simulink model "pfb_legacy"  (Simulink 6.2)
settings: Solver=ode45  StartTime=0.0  StopTime=40000  RelTol=1e-3
undefined symbols (not defined in the file): BEE2_usr
libraries: xbsIndex_r3 x189, xps_library x42, adcscope_lib x6, pfb_library x3, fft_library x3, correlator_library x3
(part 1 of 2)
settings Model: LastModifiedBy=lspitler
settings DebuggingCC: SolverPrmCheckMsg=warning

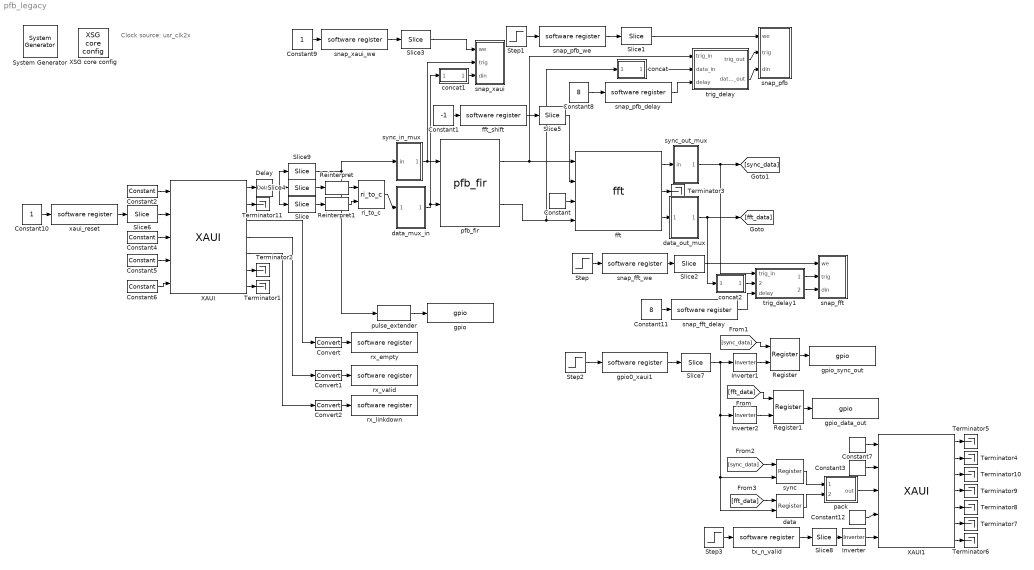
== system pfb_legacy ==
  note: Clock source: usr_clk2x
  " System Generator" : xbsIndex_r3/ System Generator  Tag=genX  xilinxfamily=Virtex2P  part=xc2vp70  speed=-7  package=ff1704  synthesis_tool=XST  directory=./pfb_legacy/sysgen  testbench=off  simulink_period=1  sysclk_period=5  incr_netlist=off  trim_vbits=Everywhere in SubSystem  dbl_ovrd=According to Block Masks  core_generation=According to Block Masks  run_coregen=off  deprecated_control=off  eval_field=0
      settings: AttributesFormatString=System\nGenerator
  Constant : xbsIndex_r3/Constant  const=0  equ=P=C  arith_type=Unsigned  n_bits=36  bin_pt=0  opselect=C  inp2=PCIN>>17  opr=+  inp1=P  carry=CIN  iostate=0  explicit_period=on  period=1  dbl_ovrd=off
  Constant1 : Constant  Value=-1
  Constant10 : Constant
  Constant11 : Constant  Value=8
  Constant12 : xbsIndex_r3/Constant  const=0  equ=P=C  arith_type=Unsigned  n_bits=4  bin_pt=0  opselect=C  inp2=PCIN>>17  opr=+  inp1=P  carry=CIN  iostate=0  explicit_period=on  period=1  dbl_ovrd=off
  Constant2 : xbsIndex_r3/Constant  const=1  equ=P=C  arith_type=Boolean  n_bits=1  bin_pt=0  opselect=C  inp2=PCIN>>17  opr=+  inp1=P  carry=CIN  iostate=0  explicit_period=on  period=1  dbl_ovrd=off
  Constant3 : xbsIndex_r3/Constant  const=0  equ=P=C  arith_type=Boolean  n_bits=36  bin_pt=0  opselect=C  inp2=PCIN>>17  opr=+  inp1=P  carry=CIN  iostate=0  explicit_period=on  period=1  dbl_ovrd=off
  Constant4 : xbsIndex_r3/Constant  const=0  equ=P=C  arith_type=Unsigned  n_bits=32  bin_pt=0  opselect=C  inp2=PCIN>>17  opr=+  inp1=P  carry=CIN  iostate=0  explicit_period=on  period=1  dbl_ovrd=off
  Constant5 : xbsIndex_r3/Constant  const=0  equ=P=C  arith_type=Unsigned  n_bits=4  bin_pt=0  opselect=C  inp2=PCIN>>17  opr=+  inp1=P  carry=CIN  iostate=0  explicit_period=on  period=1  dbl_ovrd=off
  Constant6 : xbsIndex_r3/Constant  const=0  equ=P=C  arith_type=Boolean  n_bits=1  bin_pt=0  opselect=C  inp2=PCIN>>17  opr=+  inp1=P  carry=CIN  iostate=0  explicit_period=on  period=1  dbl_ovrd=off
  Constant7 : xbsIndex_r3/Constant  const=1  equ=P=C  arith_type=Boolean  n_bits=36  bin_pt=0  opselect=C  inp2=PCIN>>17  opr=+  inp1=P  carry=CIN  iostate=0  explicit_period=on  period=1  dbl_ovrd=off
  Constant8 : Constant  Value=8
  Constant9 : Constant
  Convert : xbsIndex_r3/Convert  arith_type=Unsigned  n_bits=32  bin_pt=0  quantization=Truncate  overflow=Wrap  latency=0  explicit_period=on  period=1  dbl_ovrd=off  show_param=off  inserted_by_tool=off  pipeline=off
      settings: xl_area=[0, 0, 0, 0, 0, 0, 0]
  Convert1 : xbsIndex_r3/Convert  arith_type=Unsigned  n_bits=32  bin_pt=0  quantization=Truncate  overflow=Wrap  latency=0  explicit_period=on  period=1  dbl_ovrd=off  show_param=off  inserted_by_tool=off  pipeline=off
      settings: xl_area=[0, 0, 0, 0, 0, 0, 0]
  Convert2 : xbsIndex_r3/Convert  arith_type=Unsigned  n_bits=32  bin_pt=0  quantization=Truncate  overflow=Wrap  latency=0  explicit_period=on  period=1  dbl_ovrd=off  show_param=off  inserted_by_tool=off  pipeline=off
      settings: xl_area=[0, 0, 0, 0, 0, 0, 0]
  Delay : xbsIndex_r3/Delay  latency=1  reg_retiming=off  explicit_period=on  period=1  en=off  accept_only_valid=off  init_zero=on  dbl_ovrd=off  show_param=off
      settings: xl_area=[0, 0, 0, 0, 0, 0, 0]
  Inverter : xbsIndex_r3/Inverter  latency=0  explicit_period=off  period=1  en=off  dbl_ovrd=off  show_param=off
      settings: xl_area=[0, 0, 0, 0, 0, 0, 0]
  Inverter1 : xbsIndex_r3/Inverter  latency=0  explicit_period=off  period=1  en=off  dbl_ovrd=off  show_param=off
      settings: xl_area=[0, 0, 0, 0, 0, 0, 0]
  Inverter2 : xbsIndex_r3/Inverter  latency=0  explicit_period=off  period=1  en=off  dbl_ovrd=off  show_param=off
      settings: xl_area=[0, 0, 0, 0, 0, 0, 0]
  Register : xbsIndex_r3/Register  init=0  reg_only_valid=off  explicit_period=off  period=1  rst=off  en=on  out_en=off  dbl_ovrd=off  show_param=off
      settings: xl_area=[0, 0, 0, 0, 0, 0, 0]
  Register1 : xbsIndex_r3/Register  init=0  reg_only_valid=off  explicit_period=off  period=1  rst=off  en=on  out_en=off  dbl_ovrd=off  show_param=off
      settings: xl_area=[0, 0, 0, 0, 0, 0, 0]
  Reinterpret : xbsIndex_r3/Reinterpret  force_arith_type=on  arith_type="Signed  (2's comp)"  force_bin_pt=on  bin_pt=14  force_valid=on
  Reinterpret1 : xbsIndex_r3/Reinterpret  force_arith_type=on  arith_type="Signed  (2's comp)"  force_bin_pt=on  bin_pt=14  force_valid=on
  Slice : xbsIndex_r3/Slice  mode=Lower Bit Location + Width  nbits=15  bit1=0  base1=MSB of Input  bit0=0  base0=LSB of Input  boolean_output=off  explicit_period=on  period=1  dbl_ovrd=off
  Slice{1..3,6..8} (6 alike) : xbsIndex_r3/Slice  mode=Lower Bit Location + Width  nbits=1  bit1=0  base1=MSB of Input  bit0=0  base0=LSB of Input  boolean_output=on  explicit_period=on  period=1  dbl_ovrd=off
  Slice4 : xbsIndex_r3/Slice  mode=Lower Bit Location + Width  nbits=15  bit1=0  base1=MSB of Input  bit0=15  base0=LSB of Input  boolean_output=off  explicit_period=on  period=1  dbl_ovrd=off
  Slice5 : xbsIndex_r3/Slice  mode=Lower Bit Location + Width  nbits=12  bit1=0  base1=MSB of Input  bit0=0  base0=LSB of Input  boolean_output=off  explicit_period=off  period=1  dbl_ovrd=off
  Slice9 : xbsIndex_r3/Slice  mode=Lower Bit Location + Width  nbits=1  bit1=0  base1=MSB of Input  bit0=30  base0=LSB of Input  boolean_output=on  explicit_period=on  period=1  dbl_ovrd=off
  Step{,1..3} (4 alike) : Step  SampleTime=0
  Terminator{1..11} (11 alike) : Terminator
  XAUI : xps_library/XAUI  Tag=xps:xaui  demux=2  port=BEE2_usr:0  show_param=off  pre_emph=3  swing=800
  XAUI1 : xps_library/XAUI  Tag=xps:xaui  demux=2  port=BEE2_usr:1  show_param=off  pre_emph=3  swing=800
  XSG core config : xps_library/XSG core config  Tag=xps:xsg  hw_sys=BEE2_usr  ibob_linux=off  clk_src=usr_clk2x  gpio_clk_io_group=iBOB:sma  gpio_clk_bit_index=0  clk_rate=200  sample_period=1  synthesis_tool=XST  mpc_type=powerpc405
  concat : Subsystem
  concat1 : Subsystem
  concat2 : Subsystem
  data : xbsIndex_r3/Register  init=0  reg_only_valid=off  explicit_period=off  period=1  rst=off  en=on  out_en=off  dbl_ovrd=off  show_param=off
      settings: xl_area=[0, 0, 0, 0, 0, 0, 0]
  data_mux_in : Subsystem
  data_out_mux : Subsystem
  fft : fft_library/fft  FFTSize=12  BitWidth=18  n_inputs=0  quantization=Truncate  overflow=Wrap  add_latency=3  mult_latency=4  bram_latency=3
  fft_shift : xps_library/software register  Tag=xps:sw_reg  io_dir=From Processor  arith_type=Unsigned  bitwidth=32  bin_pt=0  sample_period=1  gw_name=pfb_legacy_fft_shift_user_data_out
  gpio : xps_library/gpio  Tag=xps:gpio  io_group=BEE2_usr:led  io_dir=out  arith_type=Boolean  bitwidth=1  bin_pt=0  bit_index=0  sample_period=1  use_single_ended=off  use_ddr=off  reg_iob=on  reg_clk_phase=0  termination=None
  gpio0_xaui1 : xps_library/software register  Tag=xps:sw_reg  io_dir=From Processor  arith_type=Unsigned  bitwidth=32  bin_pt=0  sample_period=1  gw_name=pfb_legacy_gpio0_xaui1_user_data_out
  gpio_data_out : xps_library/gpio  Tag=xps:gpio  io_group=BEE2_usr:leftlink  io_dir=out  arith_type=Unsigned  bitwidth=36  bin_pt=0  bit_index=[0:35]  sample_period=1  use_single_ended=off  use_ddr=off  reg_iob=on  reg_clk_phase=0  termination=None
  gpio_sync_out : xps_library/gpio  Tag=xps:gpio  io_group=BEE2_usr:leftlink  io_dir=out  arith_type=Boolean  bitwidth=1  bin_pt=0  bit_index=36  sample_period=1  use_single_ended=off  use_ddr=off  reg_iob=on  reg_clk_phase=0  termination=None
  pack : Subsystem
  pfb_fir : pfb_library/pfb_fir  PFBSize=12  TotalTaps=4  WindowType=hamming  n_inputs=0  MakeBiplex=off  BitWidthIn=15  BitWidthOut=18  CoeffBitWidth=8  CoeffDistMem=off  add_latency=2  mult_latency=3  bram_latency=3  quantization=Truncate  fwidth=1
      link override pol1_in1_first_tap/sync_delay/Constant: equ=P=C
      link override pol1_in1_first_tap/sync_delay/Constant1: equ=P=C
      link override pol1_in1_first_tap/sync_delay/Constant2: equ=P=C
      link override pol1_in1_first_tap/sync_delay/Constant3: equ=P=C
      link override pol1_in1_last_tap/pfb_add_tree/convert1: arith_type="Signed  (2's comp)"  n_bits=BitWidthOut  bin_pt=BitWidthOut-1  quantization=Truncate  overflow=Saturate  latency=add_latency  pipeline=on
      link override pol1_in1_last_tap/pfb_add_tree/convert2: arith_type="Signed  (2's comp)"  n_bits=BitWidthOut  bin_pt=BitWidthOut-1  quantization="Round  (unbiased: +/- Inf)"  overflow=Saturate  latency=add_latency  pipeline=on
      link override pol1_in1_tap2/sync_delay/Constant: equ=P=C
      link override pol1_in1_tap2/sync_delay/Constant1: equ=P=C
      link override pol1_in1_tap2/sync_delay/Constant2: equ=P=C
      link override pol1_in1_tap2/sync_delay/Constant3: equ=P=C
      link override pol1_in1_tap3/sync_delay/Constant: equ=P=C
      link override pol1_in1_tap3/sync_delay/Constant1: equ=P=C
      link override pol1_in1_tap3/sync_delay/Constant2: equ=P=C
      link override pol1_in1_tap3/sync_delay/Constant3: equ=P=C
      link override pol1_in2_first_tap/sync_delay/Constant: equ=P=C
      link override pol1_in2_first_tap/sync_delay/Constant1: equ=P=C
      link override pol1_in2_first_tap/sync_delay/Constant2: equ=P=C
      link override pol1_in2_first_tap/sync_delay/Constant3: equ=P=C
  pulse_extender : adcscope_lib/pulse_extender  pulse_len=2^12-1
  ri_to_c : fft_library/ri_to_c  likes_cookies=off
  rx_empty : xps_library/software register  Tag=xps:sw_reg  io_dir=To Processor  arith_type=Unsigned  bitwidth=32  bin_pt=0  sample_period=1  gw_name=pfb_legacy_rx_empty_user_data_in
  rx_linkdown : xps_library/software register  Tag=xps:sw_reg  io_dir=To Processor  arith_type=Unsigned  bitwidth=32  bin_pt=0  sample_period=1  gw_name=pfb_legacy_rx_linkdown_user_data_in
  rx_valid : xps_library/software register  Tag=xps:sw_reg  io_dir=To Processor  arith_type=Unsigned  bitwidth=32  bin_pt=0  sample_period=1  gw_name=pfb_legacy_rx_valid_user_data_in
  snap_fft : Subsystem  mask{nsamples=12}
      mask prompts: nsamples "number of samples (2^?)"
  snap_fft_delay : xps_library/software register  Tag=xps:sw_reg  io_dir=From Processor  arith_type=Unsigned  bitwidth=32  bin_pt=0  sample_period=1  gw_name=pfb_legacy_snap_fft_delay_user_data_out
  snap_fft_we : xps_library/software register  Tag=xps:sw_reg  io_dir=From Processor  arith_type=Unsigned  bitwidth=32  bin_pt=0  sample_period=1  gw_name=pfb_legacy_snap_fft_we_user_data_out
  snap_pfb : Subsystem  mask{nsamples=12}
      mask prompts: nsamples "number of samples (2^?)"
  snap_pfb_delay : xps_library/software register  Tag=xps:sw_reg  io_dir=From Processor  arith_type=Unsigned  bitwidth=32  bin_pt=0  sample_period=1  gw_name=pfb_legacy_snap_pfb_delay_user_data_out
  snap_pfb_we : xps_library/software register  Tag=xps:sw_reg  io_dir=From Processor  arith_type=Unsigned  bitwidth=32  bin_pt=0  sample_period=1  gw_name=pfb_legacy_snap_pfb_we_user_data_out
  snap_xaui : Subsystem  mask{nsamples=12}
      mask prompts: nsamples "number of samples (2^?)"
  snap_xaui_we : xps_library/software register  Tag=xps:sw_reg  io_dir=From Processor  arith_type=Unsigned  bitwidth=32  bin_pt=0  sample_period=1  gw_name=pfb_legacy_snap_xaui_we_user_data_out
  sync : xbsIndex_r3/Register  init=0  reg_only_valid=off  explicit_period=off  period=1  rst=off  en=on  out_en=off  dbl_ovrd=off  show_param=off
      settings: xl_area=[0, 0, 0, 0, 0, 0, 0]
  sync_in_mux : Subsystem
  sync_out_mux : Subsystem
  trig_delay : Subsystem
  trig_delay1 : Subsystem
  tx_n_valid : xps_library/software register  Tag=xps:sw_reg  io_dir=From Processor  arith_type=Unsigned  bitwidth=32  bin_pt=0  sample_period=1  gw_name=pfb_legacy_tx_n_valid_user_data_out
  xaui_reset : xps_library/software register  Tag=xps:sw_reg  io_dir=From Processor  arith_type=Unsigned  bitwidth=32  bin_pt=0  sample_period=1  gw_name=pfb_legacy_xaui_reset_user_data_out
  wires:
  XAUI/1 -> Delay/1
  XAUI/4 -> Convert1/1
  pfb_fir/1 -> trig_delay/1(trig_in), fft/1
  Constant2/1 -> XAUI/1
  Constant4/1 -> XAUI/3
  Constant5/1 -> XAUI/4
  Constant6/1 -> XAUI/5
  XAUI/7 -> Terminator1/1
  XAUI/6 -> Terminator2/1
  Convert/1 -> rx_empty/1
  Convert1/1 -> rx_valid/1
  Convert2/1 -> rx_linkdown/1
  XAUI/3 -> Convert/1
  XAUI/5 -> Convert2/1
  Constant/1 -> fft/3
  data_mux_in/1(Out2) -> pfb_fir/2, concat1/1(In1)
  pfb_fir/2 -> fft/4, concat/1(In1)
  fft/2 -> Terminator3/1
  fft/3 -> data_out_mux/1(In1)
  fft/1 -> sync_out_mux/1(in)
  sync_out_mux/1(out) -> trig_delay1/1(trig_in), [sync_data]
  data_out_mux/1(Out2) -> concat2/1(In1), [fft_data]
  snap_fft_we/1 -> Slice2/1
  Step/1 -> snap_fft_we/1
  snap_xaui_we/1 -> Slice3/1
  Slice3/1 -> snap_xaui/1(we)
  Constant9/1 -> snap_xaui_we/1
  Slice2/1 -> snap_fft/1(we)
  fft_shift/1 -> Slice5/1
  Constant1/1 -> fft_shift/1
  sync_in_mux/1(out) -> pfb_fir/1, snap_xaui/2(trig)
  Slice5/1 -> fft/2
  xaui_reset/1 -> Slice6/1
  Constant10/1 -> xaui_reset/1
  Slice6/1 -> XAUI/2
  concat1/1(Out1) -> snap_xaui/3(din)
  snap_pfb_we/1 -> Slice1/1
  Step1/1 -> snap_pfb_we/1
  Slice1/1 -> snap_pfb/1(we)
  pulse_extender/1 -> gpio/1
  Constant3/1 -> XAUI1/2
  Constant7/1 -> XAUI1/1
  tx_n_valid/1 -> Slice8/1
  Step3/1 -> tx_n_valid/1
  Slice8/1 -> Inverter/1
  Inverter/1 -> XAUI1/5
  XAUI1/1 -> Terminator5/1
  XAUI1/2 -> Terminator4/1
  XAUI1/6 -> Terminator7/1
  XAUI1/7 -> Terminator6/1
  XAUI1/3 -> Terminator10/1
  XAUI1/4 -> Terminator9/1
  XAUI1/5 -> Terminator8/1
  Constant8/1 -> snap_pfb_delay/1
  snap_pfb_delay/1 -> trig_delay/3(delay)
  concat/1(Out1) -> trig_delay/2(data_in)
  trig_delay/1(trig_out) -> snap_pfb/2(trig)
  trig_delay/2(data_out) -> snap_pfb/3(din)
  snap_fft_delay/1 -> trig_delay1/3(delay)
  concat2/1(Out1) -> trig_delay1/2(data_in)
  trig_delay1/1(trig_out) -> snap_fft/2(trig)
  trig_delay1/2(data_out) -> snap_fft/3(din)
  Constant11/1 -> snap_fft_delay/1
  Delay/1 -> Slice9/1, Slice4/1, Slice/1
  XAUI/2 -> Terminator11/1
  Slice9/1 -> sync_in_mux/1(in), pulse_extender/1
  Slice4/1 -> Reinterpret/1
  Slice/1 -> Reinterpret1/1
  Reinterpret/1 -> ri_to_c/1
  Reinterpret1/1 -> ri_to_c/2
  ri_to_c/1 -> data_mux_in/1(In1)
  Register/1 -> gpio_sync_out/1
  gpio0_xaui1/1 -> Slice7/1
  Slice7/1 -> Inverter1/1, Inverter2/1, sync/2, data/2
  Register1/1 -> gpio_data_out/1
  Inverter1/1 -> Register/2
  Step2/1 -> gpio0_xaui1/1
  Inverter2/1 -> Register1/2
  [fft_data] -> Register1/1
  [sync_data] -> Register/1
  pack/1(out) -> XAUI1/3
  sync/1 -> pack/1(sync)
  data/1 -> pack/2(data)
  [sync_data] -> sync/1
  [fft_data] -> data/1
  Constant12/1 -> XAUI1/4

== system pfb_legacy/concat ==
  In1 : Inport  Orientation=down  Port=1  LatchInput=off
  Concat : xbsIndex_r3/Concat  num_inputs=4  explicit_period=on  period=1  dbl_ovrd=off
  Constant7 : xbsIndex_r3/Constant  const=0  equ=P=C  arith_type=Unsigned  n_bits=14  bin_pt=0  opselect=C  inp2=PCIN>>17  opr=+  inp1=P  carry=CIN  iostate=0  explicit_period=on  period=1  dbl_ovrd=off
  Constant8 : xbsIndex_r3/Constant  const=0  equ=P=C  arith_type=Unsigned  n_bits=14  bin_pt=0  opselect=C  inp2=PCIN>>17  opr=+  inp1=P  carry=CIN  iostate=0  explicit_period=on  period=1  dbl_ovrd=off
  Slice : xbsIndex_r3/Slice  mode=Upper Bit Location + Width  nbits=18  bit1=0  base1=MSB of Input  bit0=0  base0=LSB of Input  boolean_output=off  explicit_period=on  period=1  dbl_ovrd=off
  Slice1 : xbsIndex_r3/Slice  mode=Lower Bit Location + Width  nbits=18  bit1=0  base1=MSB of Input  bit0=0  base0=LSB of Input  boolean_output=off  explicit_period=on  period=1  dbl_ovrd=off
  Out1 : Outport
  wires:
  Slice/1 -> Concat/2
  Slice1/1 -> Concat/4
  Constant7/1 -> Concat/1
  Constant8/1 -> Concat/3
  In1/1 -> Slice/1, Slice1/1
  Concat/1 -> Out1/1

== system pfb_legacy/concat1 ==
  In1 : Inport  Port=1  LatchInput=off
  Concat1 : xbsIndex_r3/Concat  num_inputs=4  explicit_period=on  period=1  dbl_ovrd=off
  Constant11 : xbsIndex_r3/Constant  const=0  equ=P=C  arith_type=Unsigned  n_bits=16  bin_pt=0  opselect=C  inp2=PCIN>>17  opr=+  inp1=P  carry=CIN  iostate=0  explicit_period=on  period=1  dbl_ovrd=off
  Constant3 : xbsIndex_r3/Constant  const=0  equ=P=C  arith_type=Unsigned  n_bits=16  bin_pt=0  opselect=C  inp2=PCIN>>17  opr=+  inp1=P  carry=CIN  iostate=0  explicit_period=on  period=1  dbl_ovrd=off
  Slice7 : xbsIndex_r3/Slice  mode=Upper Bit Location + Width  nbits=16  bit1=0  base1=MSB of Input  bit0=0  base0=LSB of Input  boolean_output=off  explicit_period=on  period=1  dbl_ovrd=off
  Slice8 : xbsIndex_r3/Slice  mode=Lower Bit Location + Width  nbits=16  bit1=0  base1=MSB of Input  bit0=0  base0=LSB of Input  boolean_output=off  explicit_period=on  period=1  dbl_ovrd=off
  Out1 : Outport
  wires:
  Slice7/1 -> Concat1/2
  Slice8/1 -> Concat1/4
  Constant3/1 -> Concat1/1
  Constant11/1 -> Concat1/3
  In1/1 -> Slice7/1, Slice8/1
  Concat1/1 -> Out1/1

== system pfb_legacy/concat2 ==
  In1 : Inport  Orientation=down  Port=1  LatchInput=off
  Concat : xbsIndex_r3/Concat  num_inputs=4  explicit_period=on  period=1  dbl_ovrd=off
  Constant7 : xbsIndex_r3/Constant  const=0  equ=P=C  arith_type=Unsigned  n_bits=14  bin_pt=0  opselect=C  inp2=PCIN>>17  opr=+  inp1=P  carry=CIN  iostate=0  explicit_period=on  period=1  dbl_ovrd=off
  Constant8 : xbsIndex_r3/Constant  const=0  equ=P=C  arith_type=Unsigned  n_bits=14  bin_pt=0  opselect=C  inp2=PCIN>>17  opr=+  inp1=P  carry=CIN  iostate=0  explicit_period=on  period=1  dbl_ovrd=off
  Slice : xbsIndex_r3/Slice  mode=Upper Bit Location + Width  nbits=18  bit1=0  base1=MSB of Input  bit0=0  base0=LSB of Input  boolean_output=off  explicit_period=on  period=1  dbl_ovrd=off
  Slice1 : xbsIndex_r3/Slice  mode=Lower Bit Location + Width  nbits=18  bit1=0  base1=MSB of Input  bit0=0  base0=LSB of Input  boolean_output=off  explicit_period=on  period=1  dbl_ovrd=off
  Out1 : Outport
  wires:
  Slice/1 -> Concat/2
  Slice1/1 -> Concat/4
  Constant7/1 -> Concat/1
  Constant8/1 -> Concat/3
  In1/1 -> Slice/1, Slice1/1
  Concat/1 -> Out1/1

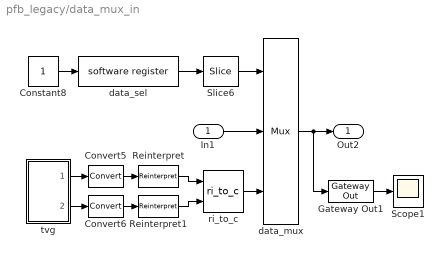
== system pfb_legacy/data_mux_in ==
  In1 : Inport  Port=1  LatchInput=off
  Constant8 : Constant
  Convert5 : xbsIndex_r3/Convert  arith_type="Signed  (2's comp)"  n_bits=15  bin_pt=0  quantization=Truncate  overflow=Wrap  latency=0  explicit_period=on  period=1  dbl_ovrd=off  show_param=off  inserted_by_tool=off  pipeline=off
      settings: xl_area=[0, 0, 0, 0, 0, 0, 0]
  Convert6 : xbsIndex_r3/Convert  arith_type="Signed  (2's comp)"  n_bits=15  bin_pt=0  quantization=Truncate  overflow=Wrap  latency=0  explicit_period=on  period=1  dbl_ovrd=off  show_param=off  inserted_by_tool=off  pipeline=off
      settings: xl_area=[0, 0, 0, 0, 0, 0, 0]
  Gateway Out1 : xbsIndex_r3/Gateway Out  output_type=Double  nbits=8  bin_pt=6  arith_type=Boolean  quantization=Truncate  overflow=Wrap  hdl_port=on  timing_constraint=None  locs_specified=off  LOCs={}  needs_fixed_name=off  show_param=off
      settings: xl_area=[0, 0, 0, 0, 0, 0, 0]
  Reinterpret : xbsIndex_r3/Reinterpret  force_arith_type=off  arith_type=Unsigned  force_bin_pt=on  bin_pt=14  force_valid=on
  Reinterpret1 : xbsIndex_r3/Reinterpret  force_arith_type=off  arith_type=Unsigned  force_bin_pt=on  bin_pt=14  force_valid=on
  Scope1 : Scope
      settings: SaveName=ScopeData5
  Slice6 : xbsIndex_r3/Slice  mode=Lower Bit Location + Width  nbits=1  bit1=0  base1=MSB of Input  bit0=0  base0=LSB of Input  boolean_output=off  explicit_period=off  period=1  dbl_ovrd=off
  data_mux : xbsIndex_r3/Mux  inputs=2  precision=Full  arith_type="Signed  (2's comp)"  n_bits=8  bin_pt=2  quantization=Truncate  overflow=Wrap  latency=0  explicit_period=on  period=1  en=off  dbl_ovrd=off  show_param=off  mux_type=off  use_rpm=off  gen_core=off
      settings: xl_area=[0, 0, 0, 0, 0, 0, 0]
  data_sel : xps_library/software register  Tag=xps:sw_reg  io_dir=From Processor  arith_type=Unsigned  bitwidth=32  bin_pt=0  sample_period=1  gw_name=pfb_legacy_data_mux_in_data_sel_user_data_out
  ri_to_c : pfb_library/tap/ri_to_c
  tvg : Subsystem
  Out2 : Outport
  wires:
  data_sel/1 -> Slice6/1
  Constant8/1 -> data_sel/1
  Slice6/1 -> data_mux/1
  In1/1 -> data_mux/2
  data_mux/1 -> Gateway Out1/1, Out2/1
  Gateway Out1/1 -> Scope1/1
  tvg/1(re_out) -> Convert5/1
  tvg/2(im_out) -> Convert6/1
  Convert5/1 -> Reinterpret/1
  Convert6/1 -> Reinterpret1/1
  ri_to_c/1 -> data_mux/3
  Reinterpret/1 -> ri_to_c/1
  Reinterpret1/1 -> ri_to_c/2

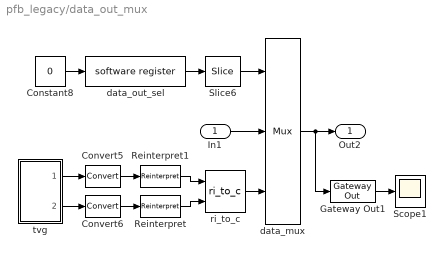
== system pfb_legacy/data_out_mux ==
  In1 : Inport  Port=1  LatchInput=off
  Constant8 : Constant  Value=0
  Convert5 : xbsIndex_r3/Convert  arith_type="Signed  (2's comp)"  n_bits=18  bin_pt=0  quantization=Truncate  overflow=Wrap  latency=0  explicit_period=on  period=1  dbl_ovrd=off  show_param=off  inserted_by_tool=off  pipeline=off
      settings: xl_area=[0, 0, 0, 0, 0, 0, 0]
  Convert6 : xbsIndex_r3/Convert  arith_type="Signed  (2's comp)"  n_bits=18  bin_pt=0  quantization=Truncate  overflow=Wrap  latency=0  explicit_period=on  period=1  dbl_ovrd=off  show_param=off  inserted_by_tool=off  pipeline=off
      settings: xl_area=[0, 0, 0, 0, 0, 0, 0]
  Gateway Out1 : xbsIndex_r3/Gateway Out  output_type=Double  nbits=8  bin_pt=6  arith_type=Boolean  quantization=Truncate  overflow=Wrap  hdl_port=on  timing_constraint=None  locs_specified=off  LOCs={}  needs_fixed_name=off  show_param=off
      settings: xl_area=[0, 0, 0, 0, 0, 0, 0]
  Reinterpret : xbsIndex_r3/Reinterpret  force_arith_type=off  arith_type=Unsigned  force_bin_pt=on  bin_pt=17  force_valid=on
  Reinterpret1 : xbsIndex_r3/Reinterpret  force_arith_type=off  arith_type=Unsigned  force_bin_pt=on  bin_pt=17  force_valid=on
  Scope1 : Scope
      settings: SaveName=ScopeData5
  Slice6 : xbsIndex_r3/Slice  mode=Lower Bit Location + Width  nbits=1  bit1=0  base1=MSB of Input  bit0=0  base0=LSB of Input  boolean_output=off  explicit_period=off  period=1  dbl_ovrd=off
  data_mux : xbsIndex_r3/Mux  inputs=2  precision=Full  arith_type="Signed  (2's comp)"  n_bits=8  bin_pt=2  quantization=Truncate  overflow=Wrap  latency=0  explicit_period=on  period=1  en=off  dbl_ovrd=off  show_param=off  mux_type=off  use_rpm=off  gen_core=off
      settings: xl_area=[0, 0, 0, 0, 0, 0, 0]
  data_out_sel : xps_library/software register  Tag=xps:sw_reg  io_dir=From Processor  arith_type=Unsigned  bitwidth=32  bin_pt=0  sample_period=1  gw_name=pfb_legacy_data_out_mux_data_out_sel_user_data_out
  ri_to_c : pfb_library/tap/ri_to_c
  tvg : Subsystem
  Out2 : Outport
  wires:
  ri_to_c/1 -> data_mux/3
  Convert6/1 -> Reinterpret/1
  tvg/2(im_out) -> Convert6/1
  tvg/1(re_out) -> Convert5/1
  Gateway Out1/1 -> Scope1/1
  data_mux/1 -> Out2/1, Gateway Out1/1
  In1/1 -> data_mux/2
  Slice6/1 -> data_mux/1
  Constant8/1 -> data_out_sel/1
  data_out_sel/1 -> Slice6/1
  Reinterpret/1 -> ri_to_c/2
  Convert5/1 -> Reinterpret1/1
  Reinterpret1/1 -> ri_to_c/1

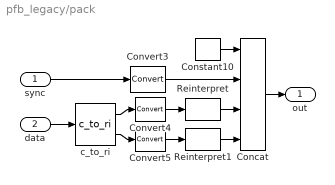
== system pfb_legacy/pack ==
  sync : Inport  Port=1  LatchInput=off
  data : Inport  Port=2  LatchInput=off
  Concat : xbsIndex_r3/Concat  num_inputs=4  explicit_period=on  period=1  dbl_ovrd=off
  Constant10 : xbsIndex_r3/Constant  const=0  equ=P=C  arith_type=Unsigned  n_bits=1  bin_pt=0  opselect=C  inp2=PCIN>>17  opr=+  inp1=P  carry=CIN  iostate=0  explicit_period=on  period=1  dbl_ovrd=off
  Convert3 : xbsIndex_r3/Convert  arith_type=Unsigned  n_bits=1  bin_pt=0  quantization=Truncate  overflow=Wrap  latency=1  explicit_period=on  period=1  dbl_ovrd=off  show_param=off  inserted_by_tool=off  pipeline=off
      settings: xl_area=[0, 0, 0, 0, 0, 0, 0]
  Convert4 : xbsIndex_r3/Convert  arith_type="Signed  (2's comp)"  n_bits=15  bin_pt=14  quantization=Truncate  overflow=Wrap  latency=1  explicit_period=on  period=1  dbl_ovrd=off  show_param=off  inserted_by_tool=off  pipeline=off
      settings: xl_area=[0, 0, 0, 0, 0, 0, 0]
  Convert5 : xbsIndex_r3/Convert  arith_type="Signed  (2's comp)"  n_bits=15  bin_pt=14  quantization=Truncate  overflow=Wrap  latency=1  explicit_period=on  period=1  dbl_ovrd=off  show_param=off  inserted_by_tool=off  pipeline=off
      settings: xl_area=[0, 0, 0, 0, 0, 0, 0]
  Reinterpret : xbsIndex_r3/Reinterpret  force_arith_type=on  arith_type=Unsigned  force_bin_pt=on  bin_pt=0  force_valid=on
  Reinterpret1 : xbsIndex_r3/Reinterpret  force_arith_type=on  arith_type=Unsigned  force_bin_pt=on  bin_pt=0  force_valid=on
  c_to_ri : fft_library/c_to_ri  BitWidth=18
  out : Outport
  wires:
  Reinterpret1/1 -> Concat/4
  Convert5/1 -> Reinterpret1/1
  data/1 -> c_to_ri/1
  Concat/1 -> out/1
  sync/1 -> Convert3/1
  Reinterpret/1 -> Concat/3
  Convert4/1 -> Reinterpret/1
  Convert3/1 -> Concat/2
  c_to_ri/2 -> Convert5/1
  c_to_ri/1 -> Convert4/1
  Constant10/1 -> Concat/1

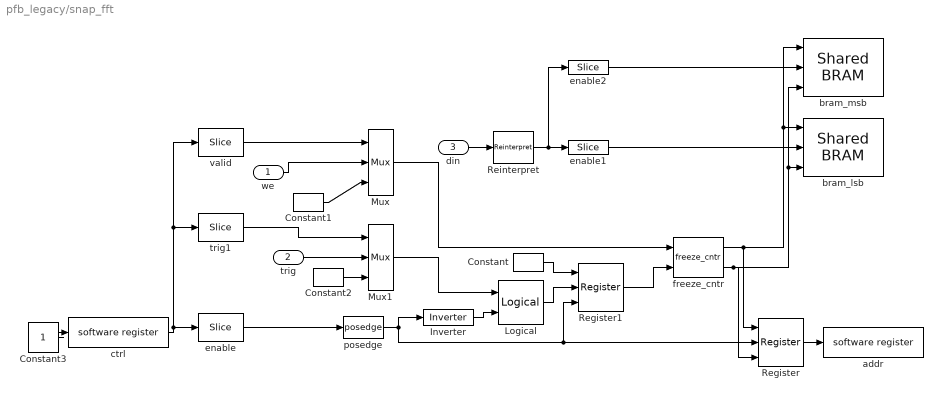
== system pfb_legacy/snap_fft ==
  we : Inport  Port=1  LatchInput=off
  trig : Inport  Port=2  LatchInput=off
  din : Inport  Port=3  LatchInput=off
  Constant : xbsIndex_r3/Constant  const=1  equ=P=C  arith_type=Boolean  n_bits=1  bin_pt=0  opselect=C  inp2=PCIN>>17  opr=+  inp1=P  carry=CIN  iostate=0  explicit_period=on  period=1  dbl_ovrd=off
  Constant1 : xbsIndex_r3/Constant  const=1  equ=P=C  arith_type=Boolean  n_bits=1  bin_pt=0  opselect=C  inp2=PCIN>>17  opr=+  inp1=P  carry=CIN  iostate=0  explicit_period=on  period=1  dbl_ovrd=off
  Constant2 : xbsIndex_r3/Constant  const=1  equ=P=C  arith_type=Boolean  n_bits=1  bin_pt=0  opselect=C  inp2=PCIN>>17  opr=+  inp1=P  carry=CIN  iostate=0  explicit_period=on  period=1  dbl_ovrd=off
  Constant3 : Constant
  Inverter : xbsIndex_r3/Inverter  latency=0  explicit_period=on  period=1  en=off  dbl_ovrd=off  show_param=off
      settings: xl_area=[0, 0, 0, 0, 0, 0, 0]
  Logical : xbsIndex_r3/Logical  logical_function=AND  inputs=2  precision=Full  arith_type=Unsigned  n_bits=8  bin_pt=2  align_bp=on  latency=0  explicit_period=off  period=1  en=off  dbl_ovrd=off  show_param=off
      settings: xl_area=[0, 0, 0, 0, 0, 0, 0]
  Mux : xbsIndex_r3/Mux  inputs=2  precision=Full  arith_type="Signed  (2's comp)"  n_bits=8  bin_pt=2  quantization=Truncate  overflow=Wrap  latency=0  explicit_period=on  period=1  en=off  dbl_ovrd=off  show_param=off  mux_type=off  use_rpm=off  gen_core=off
      settings: xl_area=[0, 0, 0, 0, 0, 0, 0]
  Mux1 : xbsIndex_r3/Mux  inputs=2  precision=Full  arith_type="Signed  (2's comp)"  n_bits=8  bin_pt=2  quantization=Truncate  overflow=Wrap  latency=0  explicit_period=on  period=1  en=off  dbl_ovrd=off  show_param=off  mux_type=off  use_rpm=off  gen_core=off
      settings: xl_area=[0, 0, 0, 0, 0, 0, 0]
  Register : xbsIndex_r3/Register  init=0  reg_only_valid=off  explicit_period=on  period=1  rst=on  en=on  out_en=off  dbl_ovrd=off  show_param=off
      settings: xl_area=[0, 0, 0, 0, 0, 0, 0]
  Register1 : xbsIndex_r3/Register  init=0  reg_only_valid=off  explicit_period=on  period=1  rst=on  en=on  out_en=off  dbl_ovrd=off  show_param=off
      settings: xl_area=[0, 0, 0, 0, 0, 0, 0]
  Reinterpret : xbsIndex_r3/Reinterpret  force_arith_type=on  arith_type=Unsigned  force_bin_pt=on  bin_pt=0  force_valid=on
  addr : xps_library/software register  Tag=xps:sw_reg  io_dir=To Processor  arith_type=Unsigned  bitwidth=32  bin_pt=0  sample_period=1  gw_name=pfb_legacy_snap_fft_addr_user_data_in
  bram_lsb : xps_library/Shared BRAM  Tag=xps:bram  arith_type=Unsigned  addr_width=nsamples  data_width=32  data_bin_pt=0  init_vals=0  sample_rate=1
  bram_msb : xps_library/Shared BRAM  Tag=xps:bram  arith_type=Unsigned  addr_width=nsamples  data_width=32  data_bin_pt=0  init_vals=0  sample_rate=1
  ctrl : xps_library/software register  Tag=xps:sw_reg  io_dir=From Processor  arith_type=Unsigned  bitwidth=32  bin_pt=0  sample_period=1  gw_name=pfb_legacy_snap_fft_ctrl_user_data_out
  enable : xbsIndex_r3/Slice  mode=Lower Bit Location + Width  nbits=1  bit1=0  base1=MSB of Input  bit0=0  base0=LSB of Input  boolean_output=on  explicit_period=on  period=1  dbl_ovrd=off
  enable1 : xbsIndex_r3/Slice  mode=Lower Bit Location + Width  nbits=32  bit1=0  base1=MSB of Input  bit0=0  base0=LSB of Input  boolean_output=off  explicit_period=on  period=1  dbl_ovrd=off
  enable2 : xbsIndex_r3/Slice  mode=Lower Bit Location + Width  nbits=32  bit1=0  base1=MSB of Input  bit0=32  base0=LSB of Input  boolean_output=off  explicit_period=on  period=1  dbl_ovrd=off
  freeze_cntr : correlator_library/freeze_cntr  CounterBits=nsamples
  posedge : adcscope_lib/posedge  Tag=Rising Edge Detector  yummy=on
  trig1 : xbsIndex_r3/Slice  mode=Lower Bit Location + Width  nbits=1  bit1=1  base1=MSB of Input  bit0=1  base0=LSB of Input  boolean_output=on  explicit_period=on  period=1  dbl_ovrd=off
  valid : xbsIndex_r3/Slice  mode=Lower Bit Location + Width  nbits=1  bit1=0  base1=MSB of Input  bit0=2  base0=LSB of Input  boolean_output=on  explicit_period=on  period=1  dbl_ovrd=off
  wires:
  Constant3/1 -> ctrl/1
  ctrl/1 -> valid/1, trig1/1, enable/1
  valid/1 -> Mux/1
  trig1/1 -> Mux1/1
  freeze_cntr/2 -> bram_msb/3, bram_lsb/3, Register/3
  freeze_cntr/1 -> Register/1, bram_msb/1, bram_lsb/1
  Mux/1 -> freeze_cntr/1
  Mux1/1 -> Logical/1
  Constant/1 -> Register1/1
  Logical/1 -> Register1/2
  Register1/1 -> freeze_cntr/2
  Inverter/1 -> Logical/2
  din/1 -> Reinterpret/1
  Constant2/1 -> Mux1/3
  Constant1/1 -> Mux/3
  trig/1 -> Mux1/2
  we/1 -> Mux/2
  Reinterpret/1 -> enable2/1, enable1/1
  enable1/1 -> bram_lsb/2
  enable2/1 -> bram_msb/2
  Register/1 -> addr/1
  posedge/1 -> Register1/3, Register/2, Inverter/1
  enable/1 -> posedge/1

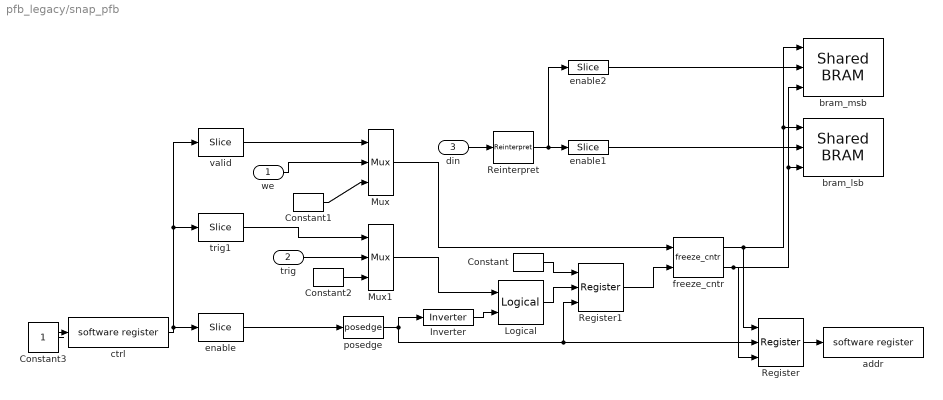
== system pfb_legacy/snap_pfb ==
  we : Inport  Port=1  LatchInput=off
  trig : Inport  Port=2  LatchInput=off
  din : Inport  Port=3  LatchInput=off
  Constant : xbsIndex_r3/Constant  const=1  equ=P=C  arith_type=Boolean  n_bits=1  bin_pt=0  opselect=C  inp2=PCIN>>17  opr=+  inp1=P  carry=CIN  iostate=0  explicit_period=on  period=1  dbl_ovrd=off
  Constant1 : xbsIndex_r3/Constant  const=1  equ=P=C  arith_type=Boolean  n_bits=1  bin_pt=0  opselect=C  inp2=PCIN>>17  opr=+  inp1=P  carry=CIN  iostate=0  explicit_period=on  period=1  dbl_ovrd=off
  Constant2 : xbsIndex_r3/Constant  const=1  equ=P=C  arith_type=Boolean  n_bits=1  bin_pt=0  opselect=C  inp2=PCIN>>17  opr=+  inp1=P  carry=CIN  iostate=0  explicit_period=on  period=1  dbl_ovrd=off
  Constant3 : Constant
  Inverter : xbsIndex_r3/Inverter  latency=0  explicit_period=on  period=1  en=off  dbl_ovrd=off  show_param=off
      settings: xl_area=[0, 0, 0, 0, 0, 0, 0]
  Logical : xbsIndex_r3/Logical  logical_function=AND  inputs=2  precision=Full  arith_type=Unsigned  n_bits=8  bin_pt=2  align_bp=on  latency=0  explicit_period=off  period=1  en=off  dbl_ovrd=off  show_param=off
      settings: xl_area=[0, 0, 0, 0, 0, 0, 0]
  Mux : xbsIndex_r3/Mux  inputs=2  precision=Full  arith_type="Signed  (2's comp)"  n_bits=8  bin_pt=2  quantization=Truncate  overflow=Wrap  latency=0  explicit_period=on  period=1  en=off  dbl_ovrd=off  show_param=off  mux_type=off  use_rpm=off  gen_core=off
      settings: xl_area=[0, 0, 0, 0, 0, 0, 0]
  Mux1 : xbsIndex_r3/Mux  inputs=2  precision=Full  arith_type="Signed  (2's comp)"  n_bits=8  bin_pt=2  quantization=Truncate  overflow=Wrap  latency=0  explicit_period=on  period=1  en=off  dbl_ovrd=off  show_param=off  mux_type=off  use_rpm=off  gen_core=off
      settings: xl_area=[0, 0, 0, 0, 0, 0, 0]
  Register : xbsIndex_r3/Register  init=0  reg_only_valid=off  explicit_period=on  period=1  rst=on  en=on  out_en=off  dbl_ovrd=off  show_param=off
      settings: xl_area=[0, 0, 0, 0, 0, 0, 0]
  Register1 : xbsIndex_r3/Register  init=0  reg_only_valid=off  explicit_period=on  period=1  rst=on  en=on  out_en=off  dbl_ovrd=off  show_param=off
      settings: xl_area=[0, 0, 0, 0, 0, 0, 0]
  Reinterpret : xbsIndex_r3/Reinterpret  force_arith_type=on  arith_type=Unsigned  force_bin_pt=on  bin_pt=0  force_valid=on
  addr : xps_library/software register  Tag=xps:sw_reg  io_dir=To Processor  arith_type=Unsigned  bitwidth=32  bin_pt=0  sample_period=1  gw_name=pfb_legacy_snap_pfb_addr_user_data_in
  bram_lsb : xps_library/Shared BRAM  Tag=xps:bram  arith_type=Unsigned  addr_width=nsamples  data_width=32  data_bin_pt=0  init_vals=0  sample_rate=1
  bram_msb : xps_library/Shared BRAM  Tag=xps:bram  arith_type=Unsigned  addr_width=nsamples  data_width=32  data_bin_pt=0  init_vals=0  sample_rate=1
  ctrl : xps_library/software register  Tag=xps:sw_reg  io_dir=From Processor  arith_type=Unsigned  bitwidth=32  bin_pt=0  sample_period=1  gw_name=pfb_legacy_snap_pfb_ctrl_user_data_out
  enable : xbsIndex_r3/Slice  mode=Lower Bit Location + Width  nbits=1  bit1=0  base1=MSB of Input  bit0=0  base0=LSB of Input  boolean_output=on  explicit_period=on  period=1  dbl_ovrd=off
  enable1 : xbsIndex_r3/Slice  mode=Lower Bit Location + Width  nbits=32  bit1=0  base1=MSB of Input  bit0=0  base0=LSB of Input  boolean_output=off  explicit_period=on  period=1  dbl_ovrd=off
  enable2 : xbsIndex_r3/Slice  mode=Lower Bit Location + Width  nbits=32  bit1=0  base1=MSB of Input  bit0=32  base0=LSB of Input  boolean_output=off  explicit_period=on  period=1  dbl_ovrd=off
  freeze_cntr : correlator_library/freeze_cntr  CounterBits=nsamples
  posedge : adcscope_lib/posedge  Tag=Rising Edge Detector  yummy=on
  trig1 : xbsIndex_r3/Slice  mode=Lower Bit Location + Width  nbits=1  bit1=1  base1=MSB of Input  bit0=1  base0=LSB of Input  boolean_output=on  explicit_period=on  period=1  dbl_ovrd=off
  valid : xbsIndex_r3/Slice  mode=Lower Bit Location + Width  nbits=1  bit1=0  base1=MSB of Input  bit0=2  base0=LSB of Input  boolean_output=on  explicit_period=on  period=1  dbl_ovrd=off
  wires:
  Constant3/1 -> ctrl/1
  ctrl/1 -> valid/1, trig1/1, enable/1
  valid/1 -> Mux/1
  trig1/1 -> Mux1/1
  freeze_cntr/2 -> bram_msb/3, bram_lsb/3, Register/3
  freeze_cntr/1 -> Register/1, bram_msb/1, bram_lsb/1
  Mux/1 -> freeze_cntr/1
  Mux1/1 -> Logical/1
  Constant/1 -> Register1/1
  Logical/1 -> Register1/2
  Register1/1 -> freeze_cntr/2
  Inverter/1 -> Logical/2
  din/1 -> Reinterpret/1
  Constant2/1 -> Mux1/3
  Constant1/1 -> Mux/3
  trig/1 -> Mux1/2
  we/1 -> Mux/2
  Reinterpret/1 -> enable2/1, enable1/1
  enable1/1 -> bram_lsb/2
  enable2/1 -> bram_msb/2
  Register/1 -> addr/1
  posedge/1 -> Register1/3, Register/2, Inverter/1
  enable/1 -> posedge/1

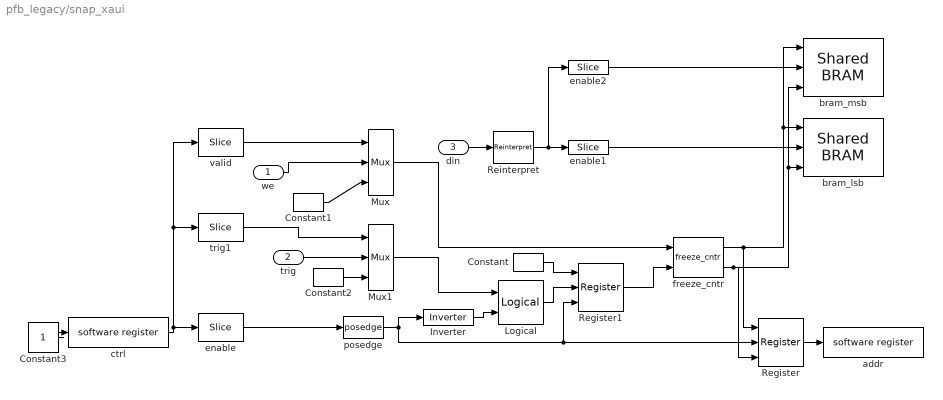
== system pfb_legacy/snap_xaui ==
  we : Inport  Port=1  LatchInput=off
  trig : Inport  Port=2  LatchInput=off
  din : Inport  Port=3  LatchInput=off
  Constant : xbsIndex_r3/Constant  const=1  equ=P=C  arith_type=Boolean  n_bits=1  bin_pt=0  opselect=C  inp2=PCIN>>17  opr=+  inp1=P  carry=CIN  iostate=0  explicit_period=on  period=1  dbl_ovrd=off
  Constant1 : xbsIndex_r3/Constant  const=1  equ=P=C  arith_type=Boolean  n_bits=1  bin_pt=0  opselect=C  inp2=PCIN>>17  opr=+  inp1=P  carry=CIN  iostate=0  explicit_period=on  period=1  dbl_ovrd=off
  Constant2 : xbsIndex_r3/Constant  const=1  equ=P=C  arith_type=Boolean  n_bits=1  bin_pt=0  opselect=C  inp2=PCIN>>17  opr=+  inp1=P  carry=CIN  iostate=0  explicit_period=on  period=1  dbl_ovrd=off
  Constant3 : Constant
  Inverter : xbsIndex_r3/Inverter  latency=0  explicit_period=on  period=1  en=off  dbl_ovrd=off  show_param=off
      settings: xl_area=[0, 0, 0, 0, 0, 0, 0]
  Logical : xbsIndex_r3/Logical  logical_function=AND  inputs=2  precision=Full  arith_type=Unsigned  n_bits=8  bin_pt=2  align_bp=on  latency=0  explicit_period=off  period=1  en=off  dbl_ovrd=off  show_param=off
      settings: xl_area=[0, 0, 0, 0, 0, 0, 0]
  Mux : xbsIndex_r3/Mux  inputs=2  precision=Full  arith_type="Signed  (2's comp)"  n_bits=8  bin_pt=2  quantization=Truncate  overflow=Wrap  latency=0  explicit_period=on  period=1  en=off  dbl_ovrd=off  show_param=off  mux_type=off  use_rpm=off  gen_core=off
      settings: xl_area=[0, 0, 0, 0, 0, 0, 0]
  Mux1 : xbsIndex_r3/Mux  inputs=2  precision=Full  arith_type="Signed  (2's comp)"  n_bits=8  bin_pt=2  quantization=Truncate  overflow=Wrap  latency=0  explicit_period=on  period=1  en=off  dbl_ovrd=off  show_param=off  mux_type=off  use_rpm=off  gen_core=off
      settings: xl_area=[0, 0, 0, 0, 0, 0, 0]
  Register : xbsIndex_r3/Register  init=0  reg_only_valid=off  explicit_period=on  period=1  rst=on  en=on  out_en=off  dbl_ovrd=off  show_param=off
      settings: xl_area=[0, 0, 0, 0, 0, 0, 0]
  Register1 : xbsIndex_r3/Register  init=0  reg_only_valid=off  explicit_period=on  period=1  rst=on  en=on  out_en=off  dbl_ovrd=off  show_param=off
      settings: xl_area=[0, 0, 0, 0, 0, 0, 0]
  Reinterpret : xbsIndex_r3/Reinterpret  force_arith_type=on  arith_type=Unsigned  force_bin_pt=on  bin_pt=0  force_valid=on
  addr : xps_library/software register  Tag=xps:sw_reg  io_dir=To Processor  arith_type=Unsigned  bitwidth=32  bin_pt=0  sample_period=1  gw_name=pfb_legacy_snap_xaui_addr_user_data_in
  bram_lsb : xps_library/Shared BRAM  Tag=xps:bram  arith_type=Unsigned  addr_width=nsamples  data_width=32  data_bin_pt=0  init_vals=0  sample_rate=1
  bram_msb : xps_library/Shared BRAM  Tag=xps:bram  arith_type=Unsigned  addr_width=nsamples  data_width=32  data_bin_pt=0  init_vals=0  sample_rate=1
  ctrl : xps_library/software register  Tag=xps:sw_reg  io_dir=From Processor  arith_type=Unsigned  bitwidth=32  bin_pt=0  sample_period=1  gw_name=pfb_legacy_snap_xaui_ctrl_user_data_out
  enable : xbsIndex_r3/Slice  mode=Lower Bit Location + Width  nbits=1  bit1=0  base1=MSB of Input  bit0=0  base0=LSB of Input  boolean_output=on  explicit_period=on  period=1  dbl_ovrd=off
  enable1 : xbsIndex_r3/Slice  mode=Lower Bit Location + Width  nbits=32  bit1=0  base1=MSB of Input  bit0=0  base0=LSB of Input  boolean_output=off  explicit_period=on  period=1  dbl_ovrd=off
  enable2 : xbsIndex_r3/Slice  mode=Lower Bit Location + Width  nbits=32  bit1=0  base1=MSB of Input  bit0=32  base0=LSB of Input  boolean_output=off  explicit_period=on  period=1  dbl_ovrd=off
  freeze_cntr : correlator_library/freeze_cntr  CounterBits=nsamples
  posedge : adcscope_lib/posedge  Tag=Rising Edge Detector  yummy=on
  trig1 : xbsIndex_r3/Slice  mode=Lower Bit Location + Width  nbits=1  bit1=1  base1=MSB of Input  bit0=1  base0=LSB of Input  boolean_output=on  explicit_period=on  period=1  dbl_ovrd=off
  valid : xbsIndex_r3/Slice  mode=Lower Bit Location + Width  nbits=1  bit1=0  base1=MSB of Input  bit0=2  base0=LSB of Input  boolean_output=on  explicit_period=on  period=1  dbl_ovrd=off
  wires:
  Constant3/1 -> ctrl/1
  ctrl/1 -> valid/1, trig1/1, enable/1
  valid/1 -> Mux/1
  trig1/1 -> Mux1/1
  freeze_cntr/2 -> bram_msb/3, bram_lsb/3, Register/3
  freeze_cntr/1 -> Register/1, bram_msb/1, bram_lsb/1
  Mux/1 -> freeze_cntr/1
  Mux1/1 -> Logical/1
  Constant/1 -> Register1/1
  Logical/1 -> Register1/2
  Register1/1 -> freeze_cntr/2
  Inverter/1 -> Logical/2
  din/1 -> Reinterpret/1
  Constant2/1 -> Mux1/3
  Constant1/1 -> Mux/3
  trig/1 -> Mux1/2
  we/1 -> Mux/2
  Reinterpret/1 -> enable2/1, enable1/1
  enable1/1 -> bram_lsb/2
  enable2/1 -> bram_msb/2
  Register/1 -> addr/1
  posedge/1 -> Register1/3, Register/2, Inverter/1
  enable/1 -> posedge/1

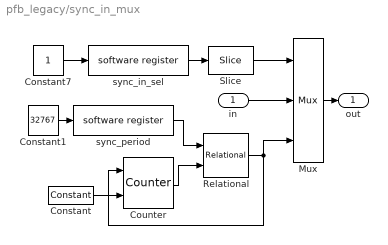
== system pfb_legacy/sync_in_mux ==
  in : Inport  Port=1  LatchInput=off
  Constant : xbsIndex_r3/Constant  const=1  equ=P=C  arith_type=Unsigned  n_bits=32  bin_pt=0  opselect=C  inp2=PCIN>>17  opr=+  inp1=P  carry=CIN  iostate=0  explicit_period=on  period=1  dbl_ovrd=off
  Constant1 : Constant  Value=32767
  Constant7 : Constant
  Counter : xbsIndex_r3/Counter  cnt_type=Free Running  n_bits=32  bin_pt=0  arith_type=Unsigned  start_count=0  cnt_to=Inf  cnt_by_val=1  operation=Up  explicit_period=on  period=1  load_pin=on  rst=off  en=off  dbl_ovrd=off  show_param=off  use_rpm=on  gen_core=off
      settings: xl_area=[0, 0, 0, 0, 0, 0, 0]
  Mux : xbsIndex_r3/Mux  inputs=2  precision=Full  arith_type="Signed  (2's comp)"  n_bits=8  bin_pt=2  quantization=Truncate  overflow=Wrap  latency=0  explicit_period=on  period=1  en=off  dbl_ovrd=off  show_param=off  mux_type=off  use_rpm=off  gen_core=off
      settings: xl_area=[0, 0, 0, 0, 0, 0, 0]
  Relational : xbsIndex_r3/Relational  mode=a=b  latency=1  explicit_period=on  period=1  en=off  dbl_ovrd=off  show_param=off
      settings: xl_area=[0, 0, 0, 0, 0, 0, 0]
  Slice : xbsIndex_r3/Slice  mode=Lower Bit Location + Width  nbits=1  bit1=0  base1=MSB of Input  bit0=0  base0=LSB of Input  boolean_output=off  explicit_period=off  period=1  dbl_ovrd=off
  sync_in_sel : xps_library/software register  Tag=xps:sw_reg  io_dir=From Processor  arith_type=Unsigned  bitwidth=32  bin_pt=0  sample_period=1  gw_name=pfb_legacy_sync_in_mux_sync_in_sel_user_data_out
  sync_period : xps_library/software register  Tag=xps:sw_reg  io_dir=From Processor  arith_type=Unsigned  bitwidth=32  bin_pt=0  sample_period=1  gw_name=pfb_legacy_sync_in_mux_sync_period_user_data_out
  out : Outport
  wires:
  Mux/1 -> out/1
  in/1 -> Mux/2
  Slice/1 -> Mux/1
  sync_in_sel/1 -> Slice/1
  Constant7/1 -> sync_in_sel/1
  Counter/1 -> Relational/2
  Relational/1 -> Counter/1, Mux/3
  sync_period/1 -> Relational/1
  Constant1/1 -> sync_period/1
  Constant/1 -> Counter/2

== system pfb_legacy/sync_out_mux ==
  in : Inport  Port=1  LatchInput=off
  Constant : xbsIndex_r3/Constant  const=1  equ=P=C  arith_type=Unsigned  n_bits=32  bin_pt=0  opselect=C  inp2=PCIN>>17  opr=+  inp1=P  carry=CIN  iostate=0  explicit_period=on  period=1  dbl_ovrd=off
  Constant1 : Constant  Value=0
  Constant7 : Constant  Value=0
  Counter : xbsIndex_r3/Counter  cnt_type=Free Running  n_bits=32  bin_pt=0  arith_type=Unsigned  start_count=0  cnt_to=Inf  cnt_by_val=1  operation=Up  explicit_period=on  period=1  load_pin=on  rst=off  en=off  dbl_ovrd=off  show_param=off  use_rpm=on  gen_core=off
      settings: xl_area=[0, 0, 0, 0, 0, 0, 0]
  Mux : xbsIndex_r3/Mux  inputs=2  precision=Full  arith_type="Signed  (2's comp)"  n_bits=8  bin_pt=2  quantization=Truncate  overflow=Wrap  latency=0  explicit_period=on  period=1  en=off  dbl_ovrd=off  show_param=off  mux_type=off  use_rpm=off  gen_core=off
      settings: xl_area=[0, 0, 0, 0, 0, 0, 0]
  Relational : xbsIndex_r3/Relational  mode=a=b  latency=1  explicit_period=on  period=1  en=off  dbl_ovrd=off  show_param=off
      settings: xl_area=[0, 0, 0, 0, 0, 0, 0]
  Slice : xbsIndex_r3/Slice  mode=Lower Bit Location + Width  nbits=1  bit1=0  base1=MSB of Input  bit0=0  base0=LSB of Input  boolean_output=off  explicit_period=off  period=1  dbl_ovrd=off
  sync_out_sel : xps_library/software register  Tag=xps:sw_reg  io_dir=From Processor  arith_type=Unsigned  bitwidth=32  bin_pt=0  sample_period=1  gw_name=pfb_legacy_sync_out_mux_sync_out_sel_user_data_out
  sync_period : xps_library/software register  Tag=xps:sw_reg  io_dir=From Processor  arith_type=Unsigned  bitwidth=32  bin_pt=0  sample_period=1  gw_name=pfb_legacy_sync_out_mux_sync_period_user_data_out
  out : Outport
  wires:
  Constant/1 -> Counter/2
  Constant1/1 -> sync_period/1
  sync_period/1 -> Relational/1
  Relational/1 -> Mux/3, Counter/1
  Counter/1 -> Relational/2
  Constant7/1 -> sync_out_sel/1
  sync_out_sel/1 -> Slice/1
  Slice/1 -> Mux/1
  in/1 -> Mux/2
  Mux/1 -> out/1

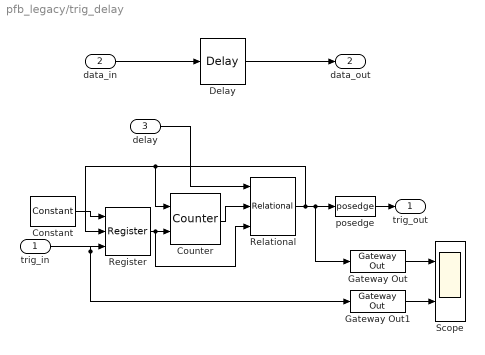
== system pfb_legacy/trig_delay ==
  trig_in : Inport  Port=1  LatchInput=off
  data_in : Inport  Port=2  LatchInput=off
  delay : Inport  Port=3  LatchInput=off
  Constant : xbsIndex_r3/Constant  const=1  equ=P=C  arith_type=Boolean  n_bits=32  bin_pt=0  opselect=C  inp2=PCIN>>17  opr=+  inp1=P  carry=CIN  iostate=0  explicit_period=on  period=1  dbl_ovrd=off
  Counter : xbsIndex_r3/Counter  cnt_type=Free Running  n_bits=32  bin_pt=0  arith_type=Unsigned  start_count=0  cnt_to=Inf  cnt_by_val=1  operation=Up  explicit_period=on  period=1  load_pin=off  rst=on  en=on  dbl_ovrd=off  show_param=off  use_rpm=on  gen_core=off
      settings: xl_area=[0, 0, 0, 0, 0, 0, 0]
  Delay : xbsIndex_r3/Delay  latency=2  reg_retiming=off  explicit_period=on  period=1  en=off  accept_only_valid=off  init_zero=on  dbl_ovrd=off  show_param=off
      settings: xl_area=[0, 0, 0, 0, 0, 0, 0]
  Gateway Out : xbsIndex_r3/Gateway Out  output_type=Double  nbits=8  bin_pt=6  arith_type=Boolean  quantization=Truncate  overflow=Wrap  hdl_port=on  timing_constraint=None  locs_specified=off  LOCs={}  needs_fixed_name=off  show_param=off
      settings: xl_area=[0, 0, 0, 0, 0, 0, 0]
  Gateway Out1 : xbsIndex_r3/Gateway Out  output_type=Double  nbits=8  bin_pt=6  arith_type=Boolean  quantization=Truncate  overflow=Wrap  hdl_port=on  timing_constraint=None  locs_specified=off  LOCs={}  needs_fixed_name=off  show_param=off
      settings: xl_area=[0, 0, 0, 0, 0, 0, 0]
  Register : xbsIndex_r3/Register  init=0  reg_only_valid=off  explicit_period=on  period=1  rst=on  en=on  out_en=off  dbl_ovrd=off  show_param=off
      settings: xl_area=[0, 0, 0, 0, 0, 0, 0]
  Relational : xbsIndex_r3/Relational  mode=a=b  latency=1  explicit_period=on  period=1  en=on  dbl_ovrd=off  show_param=off
      settings: xl_area=[0, 0, 0, 0, 0, 0, 0]
  Scope : Scope  NumInputPorts=2
      settings: YMin=-5~-5  YMax=5~5
  posedge : adcscope_lib/posedge  Tag=Rising Edge Detector  yummy=on
  trig_out : Outport
  data_out : Outport  Port=2
  wires:
  posedge/1 -> trig_out/1
  Delay/1 -> data_out/1
  data_in/1 -> Delay/1
  Gateway Out1/1 -> Scope/2
  Gateway Out/1 -> Scope/1
  Counter/1 -> Relational/2
  Register/1 -> Relational/3, Counter/2
  Relational/1 -> posedge/1, Gateway Out/1, Counter/1, Register/2
  Constant/1 -> Register/1
  trig_in/1 -> Gateway Out1/1, Register/3
  delay/1 -> Relational/1

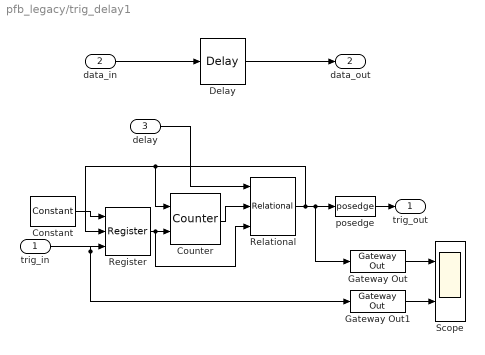
== system pfb_legacy/trig_delay1 ==
  trig_in : Inport  Port=1  LatchInput=off
  data_in : Inport  Port=2  LatchInput=off
  delay : Inport  Port=3  LatchInput=off
  Constant : xbsIndex_r3/Constant  const=1  equ=P=C  arith_type=Boolean  n_bits=32  bin_pt=0  opselect=C  inp2=PCIN>>17  opr=+  inp1=P  carry=CIN  iostate=0  explicit_period=on  period=1  dbl_ovrd=off
  Counter : xbsIndex_r3/Counter  cnt_type=Free Running  n_bits=32  bin_pt=0  arith_type=Unsigned  start_count=0  cnt_to=Inf  cnt_by_val=1  operation=Up  explicit_period=on  period=1  load_pin=off  rst=on  en=on  dbl_ovrd=off  show_param=off  use_rpm=on  gen_core=off
      settings: xl_area=[0, 0, 0, 0, 0, 0, 0]
  Delay : xbsIndex_r3/Delay  latency=2  reg_retiming=off  explicit_period=on  period=1  en=off  accept_only_valid=off  init_zero=on  dbl_ovrd=off  show_param=off
      settings: xl_area=[0, 0, 0, 0, 0, 0, 0]
  Gateway Out : xbsIndex_r3/Gateway Out  output_type=Double  nbits=8  bin_pt=6  arith_type=Boolean  quantization=Truncate  overflow=Wrap  hdl_port=on  timing_constraint=None  locs_specified=off  LOCs={}  needs_fixed_name=off  show_param=off
      settings: xl_area=[0, 0, 0, 0, 0, 0, 0]
  Gateway Out1 : xbsIndex_r3/Gateway Out  output_type=Double  nbits=8  bin_pt=6  arith_type=Boolean  quantization=Truncate  overflow=Wrap  hdl_port=on  timing_constraint=None  locs_specified=off  LOCs={}  needs_fixed_name=off  show_param=off
      settings: xl_area=[0, 0, 0, 0, 0, 0, 0]
  Register : xbsIndex_r3/Register  init=0  reg_only_valid=off  explicit_period=on  period=1  rst=on  en=on  out_en=off  dbl_ovrd=off  show_param=off
      settings: xl_area=[0, 0, 0, 0, 0, 0, 0]
  Relational : xbsIndex_r3/Relational  mode=a=b  latency=1  explicit_period=on  period=1  en=on  dbl_ovrd=off  show_param=off
      settings: xl_area=[0, 0, 0, 0, 0, 0, 0]
  Scope : Scope  NumInputPorts=2
      settings: YMin=-5~-5  YMax=5~5
  posedge : adcscope_lib/posedge  Tag=Rising Edge Detector  yummy=on
  trig_out : Outport
  data_out : Outport  Port=2
  wires:
  posedge/1 -> trig_out/1
  Delay/1 -> data_out/1
  data_in/1 -> Delay/1
  Gateway Out1/1 -> Scope/2
  Gateway Out/1 -> Scope/1
  Counter/1 -> Relational/2
  Register/1 -> Relational/3, Counter/2
  Relational/1 -> posedge/1, Gateway Out/1, Counter/1, Register/2
  Constant/1 -> Register/1
  trig_in/1 -> Gateway Out1/1, Register/3
  delay/1 -> Relational/1
